simulink model "arduino_tcpip_send_rt"  (R2023b)
settings: Solver=VariableStepDiscrete  StartTime=0.0  StopTime=inf  RelTol=1e-3
libraries: slrealtimeiplib x2
settings Model: Creator=yoany  LastModifiedBy=yoany

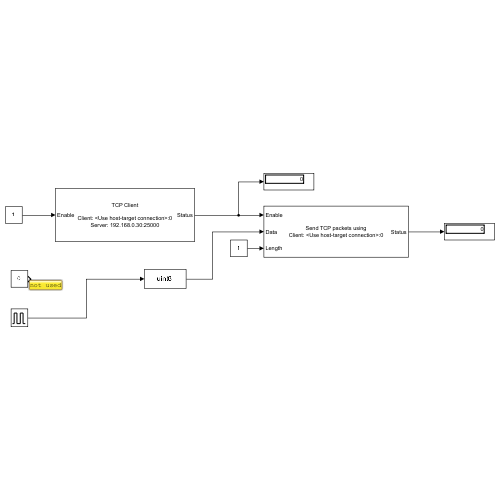
[thumbnail: Simulink's stored preview of the top-level diagram]
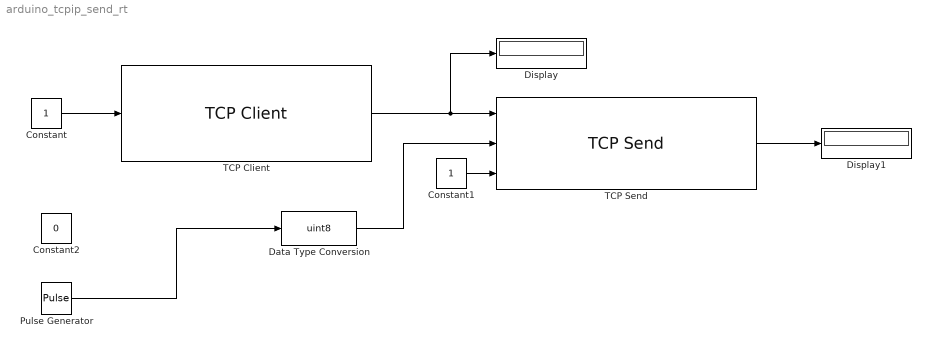
== system arduino_tcpip_send_rt ==
  Constant : Constant
  Constant1 : Constant
  Constant2 : Constant  Value=0
  Data Type Conversion : DataTypeConversion  OutDataTypeStr=uint8  SaturateOnIntegerOverflow=off  RndMeth=Floor
  Display : Display
  Display1 : Display
  Pulse Generator : DiscretePulseGenerator  PulseType=Time based  Period=10  PulseWidth=50
  TCP Client : slrealtimeiplib/TCP Client  Priority=-1  useHostTargetConn=on  remoteAddress=192.168.0.30  remotePort=25000
  TCP Send : slrealtimeiplib/TCP Send  socketAddPortVal=Client: <Use host-target connection>:0  sampleTime=0.1
  wires:
  Data Type Conversion/1 -> TCP Send/2
  TCP Client/1 -> Display/1, TCP Send/1
  Constant/1 -> TCP Client/1
  Constant1/1 -> TCP Send/3
  TCP Send/1 -> Display1/1
  Pulse Generator/1 -> Data Type Conversion/1
